simulink model "untitled"  (R2022a)
settings: Solver=VariableStepAuto  StartTime=0.0  StopTime=10  RelTol=1e-3
settings Model: Creator=Nader  LastModifiedBy=Nader

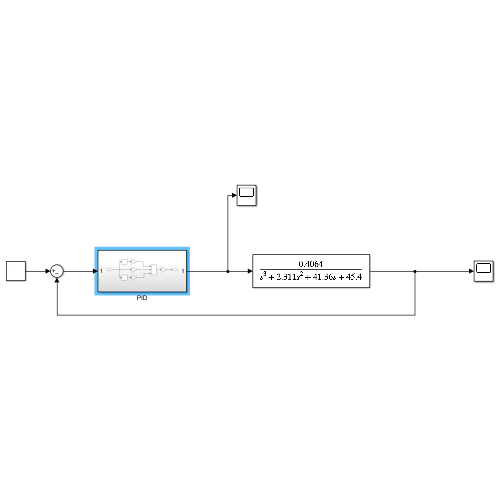
[thumbnail: Simulink's stored preview of the top-level diagram]
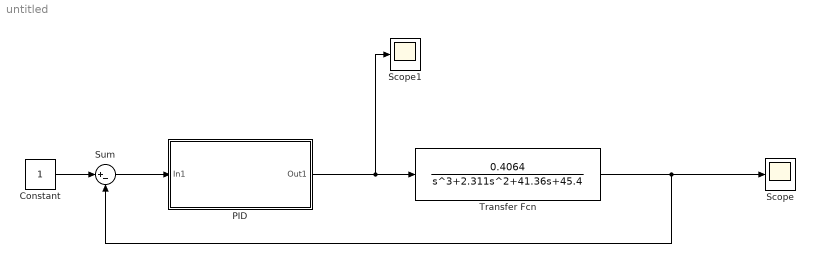
== system untitled ==
  Constant : Constant
  PID : Subsystem
  Scope : Scope
  Scope1 : Scope
  Sum : Sum  Inputs=|+-
  Transfer Fcn : TransferFcn  Numerator=0.4064  Denominator=[1, 2.311, 41.36, 45.4]
  wires:
  Transfer Fcn/1 -> Scope/1, Sum/2
  Constant/1 -> Sum/1
  Sum/1 -> PID/1(In1)
  PID/1(Out1) -> Transfer Fcn/1, Scope1/1

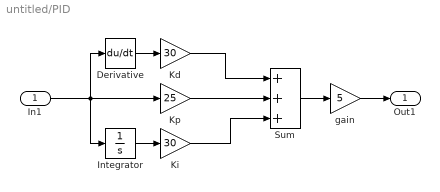
== system untitled/PID ==
  In1 : Inport
  Derivative : Derivative
  Integrator : Integrator
  Kd : Gain  Gain=30
  Ki : Gain  Gain=30
  Kp : Gain  Gain=25
  Sum : Sum  Inputs=+++
  gain : Gain  Gain=5
  Out1 : Outport
  wires:
  Derivative/1 -> Kd/1
  Integrator/1 -> Ki/1
  In1/1 -> Derivative/1, Kp/1, Integrator/1
  Kd/1 -> Sum/1
  Kp/1 -> Sum/2
  Sum/1 -> gain/1
  Ki/1 -> Sum/3
  gain/1 -> Out1/1
